simulink model "sampleModel1752_4_sub_sub"  (R2023a)
settings: Solver=VariableStepAuto  StartTime=0.0  StopTime=10.0  RelTol=1e-3
libraries: simulink x2, hdlsllib x2
settings Model: Creator=user1  LastModifiedBy=user1

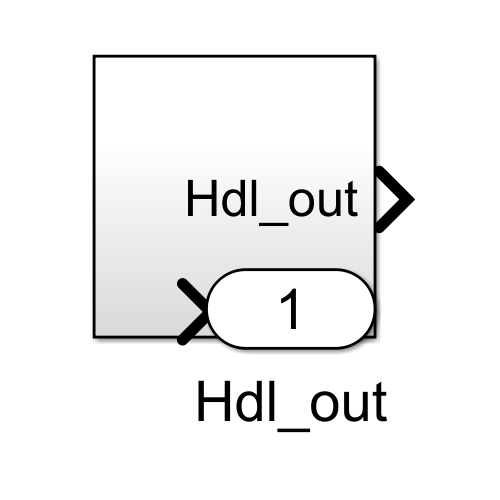
[thumbnail: Simulink's stored preview of the top-level diagram]
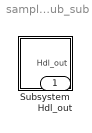
== system sampleModel1752_4_sub_sub ==
  Subsystem : Subsystem
  Hdl_out : Outport  OutDataTypeStr=uint8

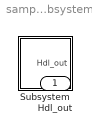
== system sampleModel1752_4_sub_sub/Subsystem ==
  Subsystem : Subsystem
  Hdl_out : Outport  OutDataTypeStr=uint8

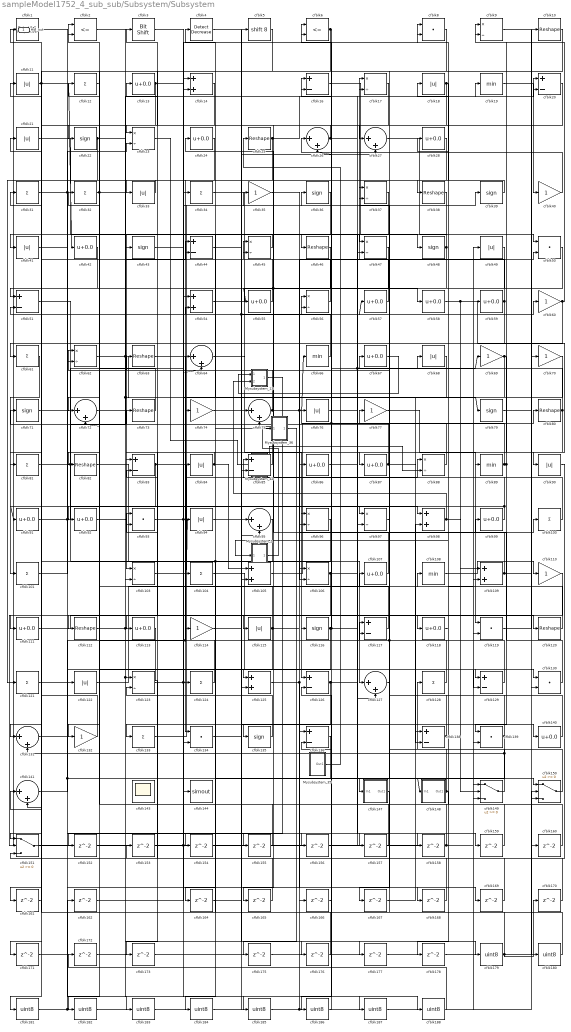
== system sampleModel1752_4_sub_sub/Subsystem/Subsystem ==
  Mysubsystem_13 : Subsystem  TreatAsAtomicUnit=on  RTWFcnName=Mysubsystem_13
      settings: RTWFcnNameOpts=User specified  RTWFileNameOpts=Use function name
  Mysubsystem_2 : Subsystem  TreatAsAtomicUnit=on  RTWFcnName=Mysubsystem_2
      settings: RTWFcnNameOpts=User specified  RTWFileNameOpts=Use function name
  Mysubsystem_35 : Subsystem  TreatAsAtomicUnit=on  RTWFcnName=Mysubsystem_35
      settings: RTWFcnNameOpts=User specified  RTWFileNameOpts=Use function name
  Mysubsystem_36 : Subsystem  TreatAsAtomicUnit=on  RTWFcnName=Mysubsystem_36
      settings: RTWFcnNameOpts=User specified  RTWFileNameOpts=Use function name
  Mysubsystem_42 : Subsystem  TreatAsAtomicUnit=on  RTWFcnName=Mysubsystem_42
      settings: RTWFcnNameOpts=User specified  RTWFileNameOpts=Use function name
  cfblk1 : hdlsllib/Logic and Bit Operations/Detect Fall Nonpositive  vinit=0  OutDataTypeStr=uint8
  cfblk{10,25,38,46,63,73,80,82,112,120} (10 alike) : Reshape
  cfblk{12,31..32,34,61,81,100..101,104,121,124,128,133} (13 alike) : Sum  Inputs=+  OutDataTypeStr=uint8
  cfblk{9,17,23,37,45,47,56,62,88,96..97,103,106,123} (14 alike) : Product  Inputs=*/  OutDataTypeStr=uint8  RndMeth=Zero  SaturateOnIntegerOverflow=on
  cfblk{14,54,98,105,109,125} (6 alike) : Sum  OutDataTypeStr=uint8
  cfblk{13,24,28,42,55,57..59,67,86..87,91..92,99,107,111,113,118,140} (19 alike) : Bias  Bias=0.0  SaturateOnIntegerOverflow=off
  cfblk{19,66,89,108} (4 alike) : MinMax  OutDataTypeStr=uint8
  cfblk{11,18,21,33,41,49,68,76,84,90,94,115,122} (13 alike) : Abs  OutDataTypeStr=uint8  SaturateOnIntegerOverflow=off
  cfblk{35,40,60,69..70,74,77,110,114,132} (10 alike) : Gain  OutDataTypeStr=uint8
  cfblk{22,36,39,43,48,71,79,116,135} (9 alike) : Signum
  cfblk{16,20,44,51,83,85,117,126,129,136,138} (11 alike) : Sum  Inputs=+-  OutDataTypeStr=uint8
  cfblk{8,50,93,119,130,134,139} (7 alike) : DotProduct  OutDataTypeStr=uint8
  cfblk{26..27,64,72,75,95,127,131,141} (9 alike) : Sum  Inputs=|++  OutDataTypeStr=uint8
  cfblk143 : Scope
      settings: Floating=on
  cfblk144 : ToWorkspace  VariableName=simout  SaveFormat=Timeseries  SampleTime=-1
  cfblk147 : Subsystem
      settings: LibrarySourceBlock=|
      | hdlsllib/Ports &
      | Subsystems/Subsystem
  cfblk148 : Subsystem
      settings: LibrarySourceBlock=|
      | hdlsllib/Ports &
      | Subsystems/Subsystem
  cfblk149 : Switch  OutDataTypeStr=uint8  SaturateOnIntegerOverflow=off  InputSameDT=off
  cfblk150 : Switch  OutDataTypeStr=uint8  SaturateOnIntegerOverflow=off  InputSameDT=off
  cfblk151 : Switch  OutDataTypeStr=uint8  SaturateOnIntegerOverflow=off  InputSameDT=off
  cfblk{152..162,164..173,175..178} (25 alike) : Delay  SampleTime=1
  cfblk{179..188} (10 alike) : DataTypeConversion  OutDataTypeStr=uint8  SaturateOnIntegerOverflow=off  RndMeth=Floor
  cfblk2 : RelationalOperator  Operator=<=  OutDataTypeStr=boolean  InputSameDT=off
  cfblk3 : hdlsllib/Logic and Bit Operations/Bit Shift  mode=Shift Left Logical  N=0
  cfblk4 : simulink/Logic and Bit Operations/Detect Decrease  vinit=0.0  OutDataTypeStr=uint8
      settings: LibrarySourceBlock=|
      | hdlsllib/Logic and Bit
      | Operations/Detect
      | Decrease
  cfblk5 : ArithShift  BitShiftNumber=8
  cfblk6 : RelationalOperator  Operator=<=  OutDataTypeStr=boolean  InputSameDT=off
  Hdl_out : Outport  OutDataTypeStr=uint8
  wires:
  Mysubsystem_42/1(Out1) -> cfblk88/2
  cfblk23/1 -> Mysubsystem_42/1(u)
  Mysubsystem_36/1(Out1) -> cfblk175/1
  Mysubsystem_2/1(Out1) -> Mysubsystem_36/1(In1)
  Mysubsystem_35/1(Out1) -> cfblk25/1
  Mysubsystem_13/1(Out1) -> cfblk152/1
  cfblk67/1 -> Mysubsystem_13/1(In1)
  cfblk188/1 -> cfblk172/1
  cfblk187/1 -> cfblk150/3
  cfblk172/1 -> cfblk187/1
  cfblk186/1 -> cfblk136/2
  cfblk185/1 -> cfblk136/1
  cfblk43/1 -> cfblk185/1
  cfblk184/1 -> cfblk166/1, cfblk49/1
  cfblk183/1 -> cfblk95/2
  cfblk182/1 -> cfblk95/1
  cfblk181/1 -> cfblk162/1, cfblk139/2
  cfblk180/1 -> cfblk4/1
  cfblk79/1 -> cfblk180/1
  cfblk179/1 -> cfblk170/1, cfblk107/1
  cfblk178/1 -> cfblk150/2
  cfblk177/1 -> cfblk109/2
  cfblk176/1 -> cfblk1/1
  cfblk175/1 -> cfblk149/3
  cfblk173/1 -> cfblk96/2
  cfblk171/1 -> cfblk119/2
  cfblk24/1 -> cfblk171/1
  cfblk170/1 -> cfblk51/2
  cfblk169/1 -> cfblk123/2
  cfblk41/1 -> cfblk169/1
  cfblk168/1 -> cfblk83/2
  cfblk167/1 -> cfblk138/1
  cfblk147/1(Out1) -> cfblk167/1
  cfblk166/1 -> cfblk126/2
  cfblk165/1 -> cfblk151/3
  cfblk164/1 -> cfblk85/2
  cfblk162/1 -> cfblk14/2
  cfblk161/1 -> cfblk141/1
  cfblk160/1 -> cfblk8/2
  cfblk9/1 -> cfblk160/1
  cfblk159/1 -> cfblk117/2
  cfblk44/1 -> cfblk159/1
  cfblk158/1 -> cfblk93/2, Hdl_out/1
  cfblk76/1 -> cfblk158/1
  cfblk157/1 -> cfblk54/1
  cfblk94/1 -> cfblk157/1
  cfblk156/1 -> cfblk98/2
  cfblk131/1 -> cfblk156/1
  cfblk155/1 -> cfblk2/2
  cfblk50/1 -> cfblk155/1
  cfblk154/1 -> cfblk97/2
  cfblk153/1 -> cfblk149/1
  cfblk90/1 -> cfblk153/1
  cfblk152/1 -> cfblk47/2
  cfblk91/1 -> cfblk43/1, cfblk125/2
  cfblk97/1 -> cfblk77/1
  cfblk74/1 -> cfblk5/1, cfblk57/1
  cfblk101/1 -> cfblk23/2
  cfblk109/1 -> cfblk70/1, cfblk45/2
  cfblk127/1 -> cfblk67/1
  cfblk115/1 -> cfblk76/1, cfblk60/1, cfblk44/1, cfblk182/1
  cfblk134/1 -> cfblk27/2
  cfblk139/1 -> cfblk63/1, cfblk164/1
  cfblk18/1 -> cfblk55/1, cfblk125/1, cfblk38/1
  cfblk26/1 -> cfblk22/1, cfblk20/1
  cfblk49/1 -> cfblk147/1(In1)
  cfblk3/1 -> cfblk98/1
  cfblk148/1(Out1) -> cfblk37/1, cfblk178/1
  cfblk130/1 -> cfblk99/1
  cfblk13/1 -> cfblk8/1, cfblk92/1
  cfblk12/1 -> cfblk72/1
  cfblk114/1 -> cfblk140/1
  cfblk25/1 -> cfblk17/2, cfblk105/2
  cfblk5/1 -> cfblk23/1
  cfblk107/1 -> cfblk24/1
  cfblk72/1 -> cfblk16/2
  cfblk80/1 -> cfblk6/1, cfblk113/1
  cfblk119/1 -> cfblk10/1
  cfblk116/1 -> cfblk19/1, cfblk56/1, cfblk165/1
  cfblk55/1 -> cfblk45/1
  cfblk85/1 -> cfblk54/2
  cfblk71/1 -> cfblk34/1
  cfblk86/1 -> cfblk120/1
  cfblk92/1 -> cfblk129/1
  cfblk121/1 -> cfblk114/1
  cfblk100/1 -> cfblk16/1
  cfblk40/1 -> cfblk26/1
  cfblk123/1 -> cfblk130/2
  cfblk1/1 -> cfblk150/1
  cfblk22/1 -> cfblk123/1, cfblk188/1, cfblk79/1, cfblk62/2
  cfblk108/1 -> cfblk110/1
  cfblk2/1 -> cfblk47/1
  cfblk69/1 -> cfblk116/1, cfblk89/1
  cfblk31/1 -> cfblk127/2, cfblk183/1
  cfblk89/1 -> cfblk139/1, cfblk9/2, cfblk6/2
  cfblk45/1 -> cfblk41/1
  cfblk84/1 -> cfblk83/1, cfblk105/1
  cfblk4/1 -> cfblk179/1
  cfblk59/1 -> cfblk13/1, cfblk112/1
  cfblk19/1 -> cfblk40/1
  cfblk150/1 -> cfblk117/1
  cfblk39/1 -> cfblk33/1
  cfblk95/1 -> cfblk181/1
  cfblk141/1 -> cfblk122/1, cfblk148/1(In1)
  cfblk135/1 -> cfblk3/1
  cfblk73/1 -> cfblk12/1
  cfblk46/1 -> cfblk103/2
  cfblk17/1 -> cfblk75/2
  cfblk129/1 -> cfblk94/1, cfblk37/2
  cfblk125/1 -> cfblk100/1, cfblk168/1
  cfblk48/1 -> cfblk46/1, cfblk131/1
  cfblk136/1 -> cfblk184/1
  cfblk112/1 -> cfblk84/1, cfblk177/1
  cfblk113/1 -> cfblk133/1
  cfblk122/1 -> cfblk59/1
  cfblk81/1 -> cfblk14/1, cfblk104/1
  cfblk6/1 -> cfblk82/1, cfblk186/1
  cfblk8/1 -> cfblk87/1
  cfblk140/1 -> cfblk28/1
  cfblk120/1 -> cfblk18/1
  cfblk36/1 -> cfblk74/1
  cfblk37/1 -> cfblk115/1
  cfblk96/1 -> cfblk141/2, cfblk154/1
  cfblk64/1 -> cfblk138/2
  cfblk10/1 -> cfblk81/1
  cfblk32/1 -> cfblk72/2, cfblk176/1
  cfblk106/1 -> cfblk151/2, cfblk68/1
  cfblk124/1 -> cfblk64/1, cfblk32/1
  cfblk56/1 -> cfblk21/1
  cfblk103/1 -> cfblk39/1
  cfblk110/1 -> cfblk151/1
  cfblk77/1 -> cfblk119/1
  cfblk138/1 -> Mysubsystem_2/1(In1), cfblk71/1
  cfblk42/1 -> cfblk51/1
  cfblk128/1 -> cfblk93/1
  cfblk60/1 -> cfblk9/1, cfblk161/1
  cfblk27/1 -> cfblk50/1
  cfblk20/1 -> cfblk27/1
  cfblk58/1 -> cfblk90/1, cfblk109/1
  cfblk70/1 -> cfblk96/1
  cfblk54/1 -> cfblk58/1
  cfblk62/1 -> cfblk144/1, cfblk44/2
  cfblk75/1 -> cfblk62/1, cfblk50/2
  cfblk126/1 -> cfblk69/1, cfblk20/2, cfblk173/1
  cfblk98/1 -> Mysubsystem_13/2(In2), cfblk149/2
  cfblk83/1 -> cfblk106/2, cfblk132/1
  cfblk117/1 -> cfblk2/1
  cfblk104/1 -> cfblk130/1
  cfblk93/1 -> cfblk88/1, cfblk35/1
  cfblk51/1 -> cfblk97/1
  cfblk151/1 -> cfblk64/2, cfblk124/1, cfblk75/1
  cfblk35/1 -> cfblk106/1
  cfblk21/1 -> cfblk86/1
  cfblk87/1 -> cfblk73/1, cfblk129/2
  cfblk11/1 -> cfblk42/1, cfblk61/1
  cfblk34/1 -> cfblk126/1
  cfblk68/1 -> cfblk134/2
  cfblk63/1 -> cfblk36/1
  cfblk111/1 -> cfblk118/1
  cfblk47/1 -> cfblk135/1
  cfblk14/1 -> cfblk111/1
  cfblk28/1 -> cfblk134/1
  cfblk57/1 -> cfblk17/1
  cfblk66/1 -> cfblk11/1
  cfblk82/1 -> cfblk127/1
  cfblk33/1 -> cfblk121/1
  cfblk16/1 -> cfblk48/1
  cfblk105/1 -> cfblk80/1
  cfblk99/1 -> cfblk91/1, cfblk56/2
  cfblk149/1 -> cfblk128/1, cfblk131/2
  cfblk38/1 -> cfblk103/1
  cfblk118/1 -> cfblk85/1
  cfblk133/1 -> cfblk108/1
  cfblk132/1 -> cfblk31/1
  cfblk88/1 -> cfblk66/1, cfblk26/2
  cfblk61/1 -> cfblk101/1

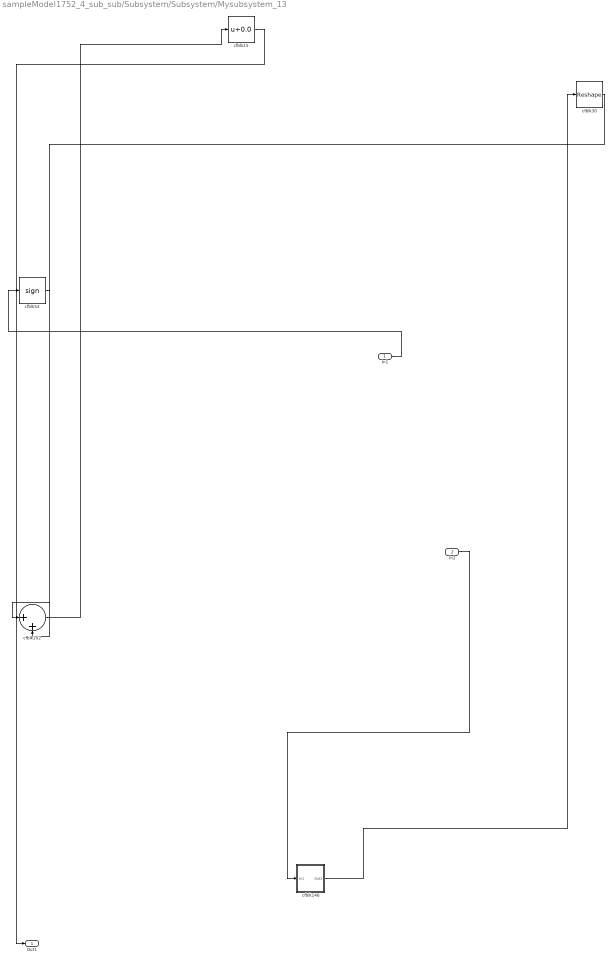
== system sampleModel1752_4_sub_sub/Subsystem/Subsystem/Mysubsystem_13 ==
  In1 : Inport
  In2 : Inport  Port=2
  cfblk102 : Sum  Inputs=|++
  cfblk146 : Subsystem
      settings: LibrarySourceBlock=|
      | hdlsllib/Ports &
      | Subsystems/Subsystem
  cfblk15 : Bias  Bias=0.0  SaturateOnIntegerOverflow=off
  cfblk30 : Reshape
  cfblk52 : Signum
  Out1 : Outport
  wires:
  In1/1 -> cfblk52/1
  cfblk30/1 -> cfblk102/2
  cfblk52/1 -> cfblk102/1
  cfblk146/1(Out1) -> cfblk30/1
  In2/1 -> cfblk146/1(In1)
  cfblk15/1 -> Out1/1
  cfblk102/1 -> cfblk15/1

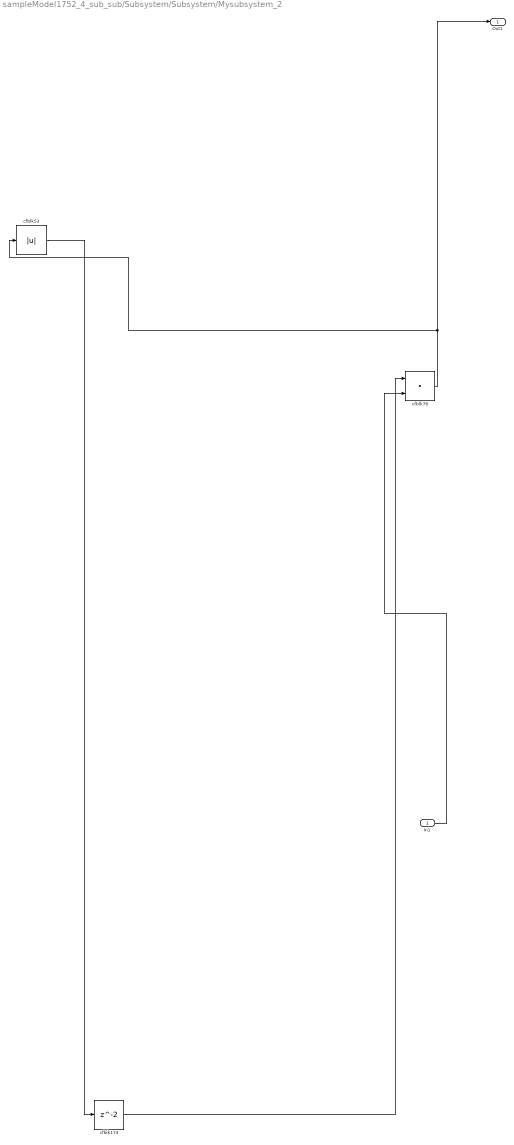
== system sampleModel1752_4_sub_sub/Subsystem/Subsystem/Mysubsystem_2 ==
  In1 : Inport
  cfblk174 : Delay  SampleTime=1
  cfblk53 : Abs  SaturateOnIntegerOverflow=off
  cfblk78 : DotProduct  OutDataTypeStr=Inherit: Inherit via internal rule
  Out1 : Outport
  wires:
  cfblk78/1 -> Out1/1, cfblk53/1
  cfblk174/1 -> cfblk78/1
  cfblk53/1 -> cfblk174/1
  In1/1 -> cfblk78/2

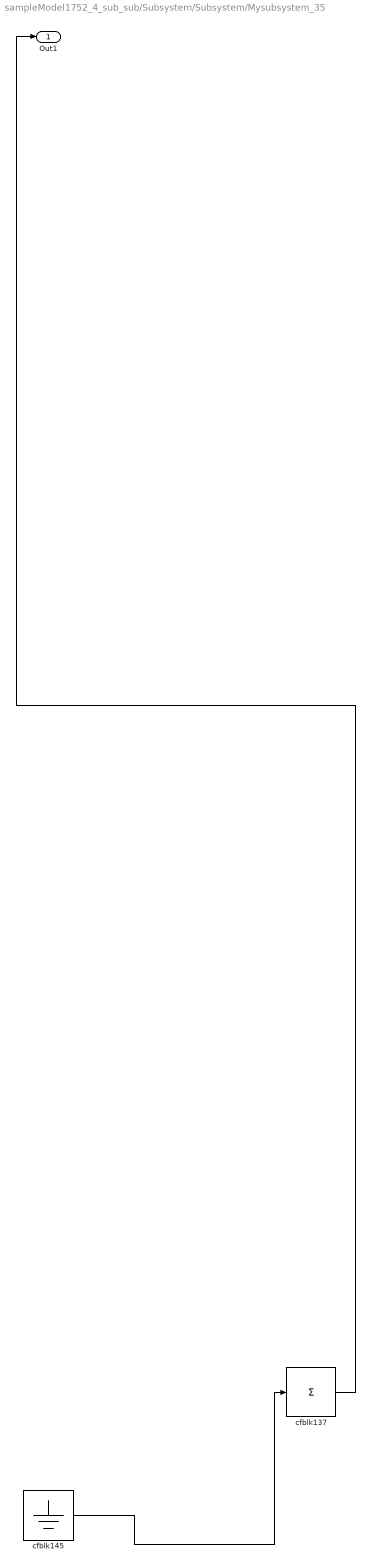
== system sampleModel1752_4_sub_sub/Subsystem/Subsystem/Mysubsystem_35 ==
  cfblk137 : Sum  Inputs=+
  cfblk145 : Ground
  Out1 : Outport
  wires:
  cfblk145/1 -> cfblk137/1
  cfblk137/1 -> Out1/1

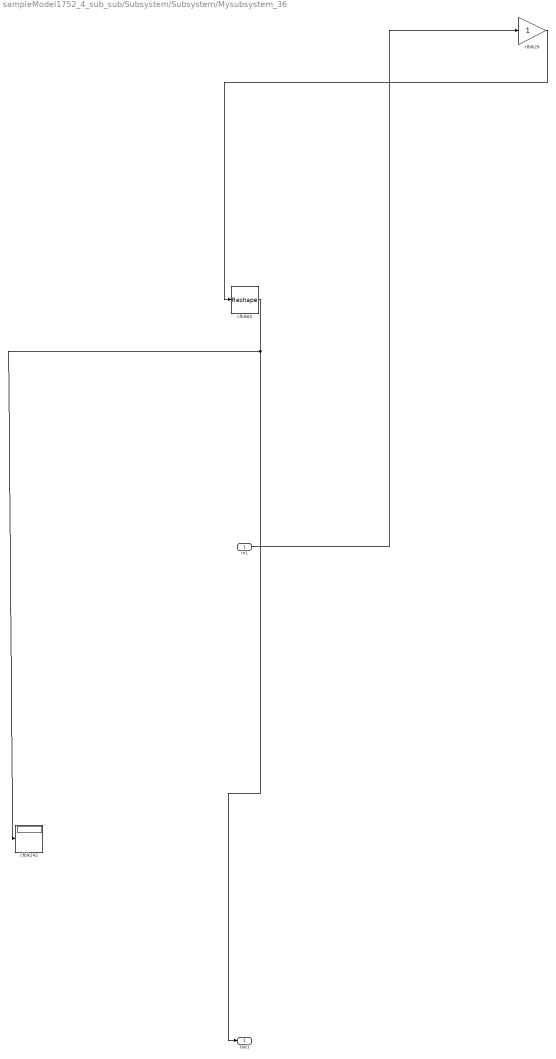
== system sampleModel1752_4_sub_sub/Subsystem/Subsystem/Mysubsystem_36 ==
  In1 : Inport
  cfblk142 : Display
  cfblk29 : Gain
  cfblk65 : Reshape
  Out1 : Outport
  wires:
  In1/1 -> cfblk29/1
  cfblk29/1 -> cfblk65/1
  cfblk65/1 -> Out1/1, cfblk142/1

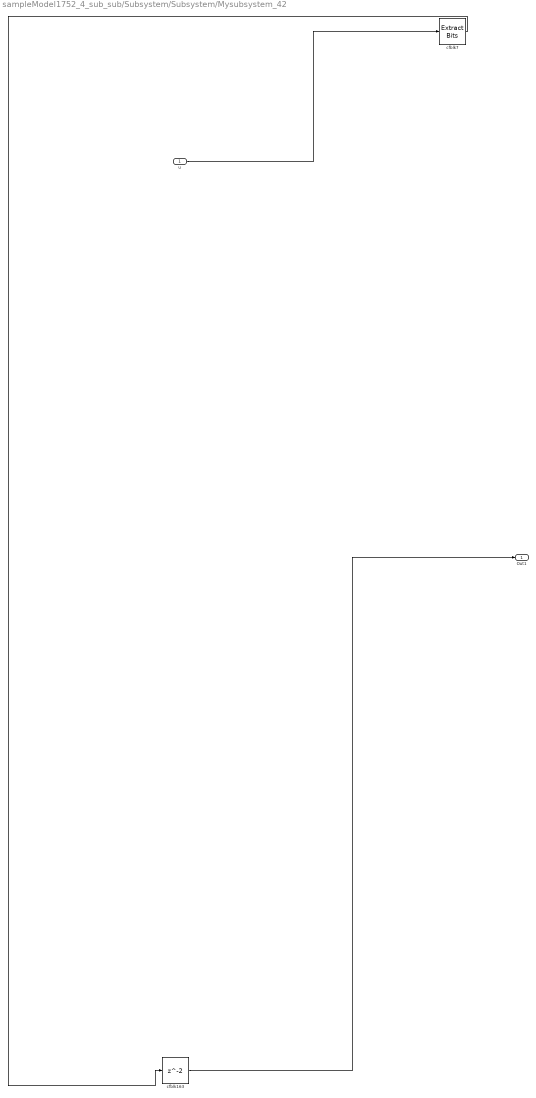
== system sampleModel1752_4_sub_sub/Subsystem/Subsystem/Mysubsystem_42 ==
  u : Inport
  cfblk163 : Delay  SampleTime=1
  cfblk7 : simulink/Logic and Bit Operations/Extract Bits  bitsToExtract=Upper half  numBits=8  bitIdxRange=[0 7]  outScalingMode=Preserve fixed-point scaling
      settings: LibrarySourceBlock=|
      | hdlsllib/Logic and Bit
      | Operations/Extract Bits
  Out1 : Outport
  wires:
  cfblk7/1 -> cfblk163/1
  u/1 -> cfblk7/1
  cfblk163/1 -> Out1/1

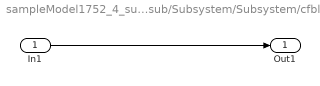
== system sampleModel1752_4_sub_sub/Subsystem/Subsystem/cfblk147 ==
  In1 : Inport
  Out1 : Outport
  wires:
  In1/1 -> Out1/1

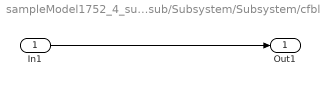
== system sampleModel1752_4_sub_sub/Subsystem/Subsystem/cfblk148 ==
  In1 : Inport
  Out1 : Outport
  wires:
  In1/1 -> Out1/1

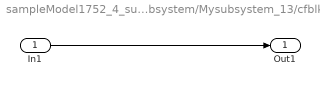
== system sampleModel1752_4_sub_sub/Subsystem/Subsystem/Mysubsystem_13/cfblk146 ==
  In1 : Inport
  Out1 : Outport
  wires:
  In1/1 -> Out1/1
